simulink model "AD_motor_test"  (R2017a)
settings: Solver=FixedStepDiscrete  StartTime=0.0  StopTime=10.0  FixedStep=100e-6  MaxStep=1e-4  RelTol=1e-3
libraries: powerlib x5, eltreclib x1
settings Model: Creator=mayartmal  LastModifiedBy=mayartmal

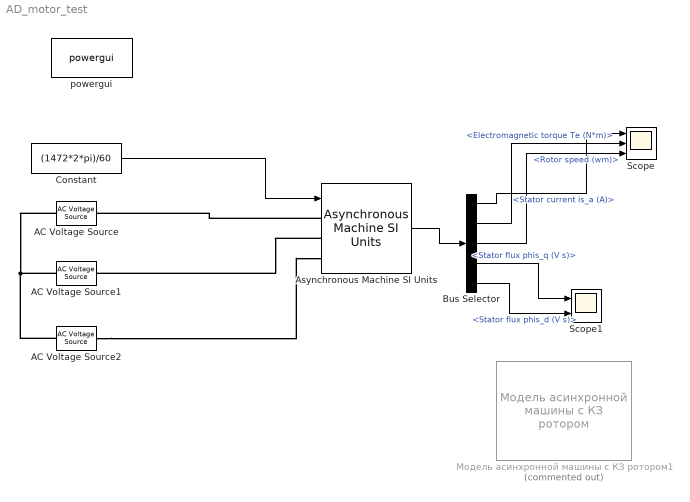
== system AD_motor_test ==
  AC Voltage Source : powerlib/Electrical Sources/AC Voltage Source  Amplitude=1293*sqrt(2)  Phase=0  Frequency=49.4  SampleTime=0  Measurements=None  BusType=swing  Pref=10e3  Qref=0  Qmin=-inf  Qmax=+inf
  AC Voltage Source1 : powerlib/Electrical Sources/AC Voltage Source  Amplitude=1293*sqrt(2)  Phase=-120  Frequency=49.4  SampleTime=0  Measurements=None  BusType=swing  Pref=10e3  Qref=0  Qmin=-inf  Qmax=+inf
  AC Voltage Source2 : powerlib/Electrical Sources/AC Voltage Source  Amplitude=1293*sqrt(2)  Phase=-240  Frequency=49.4  SampleTime=0  Measurements=None  BusType=swing  Pref=10e3  Qref=0  Qmin=-inf  Qmax=+inf
  Asynchronous Machine SI Units : powerlib/Machines/Asynchronous Machine SI Units  RotorType=Squirrel-cage  PresetModel=No  MechanicalLoad=Speed w  ShowDetailedParameters=on  ReferenceFrame=Rotor  Units=SI  MeasurementBus=off  NominalParameters=[1050000 2240 49.4]  Stator=[0.025 0.0005]  Rotor=[0.027 0.001]  Cage1=[0.4155 0.002066]  Cage2=[0.4168 0.0003495]  Lm=0.027  Mechanical=[0.05 0.005879 2]  PolePairs=2  InitialConditions=[0 0 0 0 0 0 0 0]  SimulateSaturation=off  Saturation=[14.03593122, 27.81365428, 53.79336849, 72.68890987, 97.98006896, 148.6815601, 215.7428561, 302.9841135, 428.7778367 ; 230, 322, 414, 460, 506, 552, 598, 644, 690]  LoadFlowParameters=1492000  TsPowergui=0  TsBlock=-1  IterativeModel=Trapezoidal non iterative  IterativeDiscreteModel=Trapezoidal non iterative  Pmec=1.492e+006
  Bus Selector : BusSelector  OutputSignals=Stator measurements.Stator current is_a (A),Mechanical.Electromagnetic torque Te (N*m),Mechanical.Rotor speed (wm),Stator measurements.Stator flux phis_q (V s),Stator measurements.Stator flux phis_d (V s)
  Constant : Constant  Value=(1472*2*pi)/60
  Scope : Scope  NumInputPorts=3
  Scope1 : Scope  NumInputPorts=2
  powergui : powerlib/powergui  Priority=1  SimulationMode=Discrete  SampleTime=100e-6  frequency=60  Iterations=50  frequencyindice=49.4  Pbase=100e6  ErrMax=1e-4  UnitsV=kV  UnitsW=MW  buscounter=0  FunctionMessages=off  echomessages=off  EnableUseOfTLC=off  CurrentSourceSwitches=off  DisableSnubberDevices=off  DisableRonSwitches=off  DisableVfSwitches=off  DisplayEquations=off  SolverType=Tustin/Backward Euler (TBE)  Interpol=off  ExternalGateDelay=off  methode=off  Ts=100  x0status=blocks  SPID=on  SwTol=0  HookPort=off  RestoreLinks=warning  ResistiveCurrentMeasurement=off  Frange=[0:2:500]  Ylog=off  Xlog=on  ShowGrid=off  save=off  variable=ZData  structure=0  ZoomFFT=off  StartTime=0.0  cycles=1  DisplayStyle=1  fundamental=60  FreqAxis=off  MaxFrequency=1000  frequencyindicesteady=1  RmsSteady=1  display=off
  Модель асинхронной машины с КЗ ротором1 : eltreclib/Модель асинхронной машины с КЗ ротором  Commented=on  f_nominal=50  Rs=0.025  ls=0.0005  Rr=0.027  lr=0.001  Lm=0.027  Zp=2
      settings: SourceProductName=Electric Traction
  wires:
  Constant/1 -> Asynchronous Machine SI Units/1
  Asynchronous Machine SI Units/1 -> Bus Selector/1
  Bus Selector/1 -> Scope/1  "<Stator current is_a (A)>"
  Bus Selector/2 -> Scope/2  "<Electromagnetic torque Te (N*m)>"
  Bus Selector/3 -> Scope/3  "<Rotor speed (wm)>"
  Bus Selector/5 -> Scope1/2  "<Stator flux phis_d (V s)>"
  Bus Selector/4 -> Scope1/1  "<Stator flux phis_q (V s)>"
  connections:
  AC Voltage Source/LConn1 -- AC Voltage Source2/LConn1 -- AC Voltage Source1/LConn1
  Asynchronous Machine SI Units/LConn1 -- AC Voltage Source/RConn1
  Asynchronous Machine SI Units/LConn2 -- AC Voltage Source1/RConn1
  AC Voltage Source2/RConn1 -- Asynchronous Machine SI Units/LConn3
